simulink library "tqd"  (R2021b)
settings: Solver=VariableStepAuto  StartTime=0.0  StopTime=10.0  RelTol=1e-3
undefined symbols (not defined in the file): ATQD_AfterTqMinGain_X_Deg, ATQD_APSCreepBaseTqD_X_kph, ATQD_APSCreepBaseTqD_Y_Deg, ATQD_APSCreepBaseTqR_X_kph, ATQD_APSCreepBaseTqR_Y_Deg, ATQD_APSCreepIterm_X_kph, ATQD_APSCreepIterm_Y_kph, ATQD_APSCreepPterm_X_kph, ATQD_APSCreepPterm_Y_kph, ATQD_APSDecReq_X_kph, ATQD_APSDecReq_Y_mps2, ATQD_APSDecReqCMD_X_kph, ATQD_APSDecReqTs_X_pct, ATQD_APSDecTimeGain_X_Deg, ATQD_APSDecTimeGain_Y_s, ATQD_APSReqLowSpd_X_Deg, ATQD_AutoHoldReleaseBPS_X_Deg, ATQD_AWDLoadTrqnsGain_X_kg, ATQD_AWDLoadTrqnsGain_Y_pct, ATQD_BOSEnBPSPosn_X_kph, ATQD_BOSMap_X_rpm, ATQD_BOSMap_Y_pct, ATQD_CreepBaseTqD_X_kph, ATQD_CreepBaseTqD_Y_Deg, ATQD_CreepBaseTqR_X_kph, ATQD_CreepBaseTqR_Y_Deg, ATQD_CreepBPSDisPosn_X_Deg, ATQD_CreepBPSDisPosnR_X_Deg, ATQD_CreepBPSEnPosn_X_Deg, ATQD_CreepBPSEnPosnR_X_Deg, ATQD_CreepDeltaTq_X_kph, ATQD_CreepIterm_X_kph, ATQD_CreepIterm_Y_kph, ATQD_CreepItermMaxLimit_X_pct, ATQD_CreepPreloadTime_X_kph, ATQD_CreepPreloadTq_X_kph, ATQD_CreepPreloadTq_Y_s, ATQD_CreepProtTq_X_Deg, ATQD_CreepPterm_X_kph, ATQD_CreepPterm_Y_kph, ATQD_CreepRrTqSpRat_X_rpm, ATQD_CreepRrTqSpRat_Y_Nm, ATQD_CreepTargetSpdD_X_pct, ATQD_CreepTargetSpdR_X_pct, ATQD_ECOTqMapD_X_rpm, ATQD_ECOTqMapD_Y_pct, ATQD_EMTqMapD_X_rpm, ATQD_EMTqMapD_Y_pct, ATQD_EOPDTqMapDCon_X_rpm, ATQD_EOPDTqMapDCon_Y_Deg, ATQD_EscapeModePedTq_X_pct, ATQD_EscapeModePedTq_Y_rpm, ATQD_EscapeModePedTqFr_X_pct, ATQD_EscapeModePedTqFr_Y_rpm, ATQD_EstInitVehWeight_X_c, ATQD_FAfterTqCMDGain_X_rpm, ATQD_FAfterTqCMDGain_Y_pct, ATQD_FrLossMAPLowV_X_rpm, ATQD_FrLossMAPLowV_Y_Nm, ATQD_FrMotActReduce_X_rpm ... (+772)
libraries: simulink x211, hcu_lib x179, tqr x3
(part 24 of 28)

== system tqd/TQD/TorqueDemand/TorqueModule/DriverWhlTqDem/PedalMapWhlTq/NoLHM/ShiftD/LUT_D_ECO ==
  VTQD_TqTargetShaftSpd_rpm : Inport
  VTQD_ActAPSPosn_pct : Inport  Port=2
  VTQD_RegenMode_enum : Inport  Port=3
  VTQD_RollRegenEnable_flg : Inport  Port=4
  VTQD_RollingShaftSpd_rpm : Inport  Port=5
  VVMC_EstSlope_Deg : Inport  Port=6
  VTQD_APSReqTimer_s : Inport  Port=7
  VTQD_LowIdleAccPedal_flg : Inport  Port=8
  VTQD_OPDHoldEnRel_flg : Inport  Port=9
  VTQD_OPDHoldActRelTq_Nm : Inport  Port=10
  VTQD_VehActSpd_kph : Inport  Port=11
  VTQD_SlopeUp_flg : Inport  Port=12
  RegenTqMapDComp_bus : Inport  Port=13
  Action Port : ActionPort
  Bus Selector : BusSelector  OutputSignals=VTQD_RL1TqMapDComp_Nm,VTQD_RL2TqMapDComp_Nm,VTQD_RL3TqMapDComp_Nm,VTQD_RL4TqMapDComp_Nm,VTQD_RL5TqMapDComp_Nm
  Constant : Constant  Value=ENUM_REGENLEVEL_LV1
  Constant1 : Constant  Value=ENUM_REGENLEVEL_LV2
  Constant2 : Constant  Value=ENUM_REGENLEVEL_LV3
  Constant3 : Constant  Value=ENUM_REGENLEVEL_LV4
  Constant4 : Constant  Value=ENUM_REGENLEVEL_LV5
  Constant5 : Constant  Value=ENUM_REGENLEVEL_OPD
  ECO_Invalid_TqMap1 : Subsystem  TreatAsAtomicUnit=on
  ECO_Lv1_TqMap : Subsystem  TreatAsAtomicUnit=on
  ECO_Lv2_TqMap : Subsystem  TreatAsAtomicUnit=on
  ECO_Lv3_TqMap : Subsystem  TreatAsAtomicUnit=on
  ECO_Lv4_TqMap : Subsystem  TreatAsAtomicUnit=on
  ECO_Lv5_TqMap : Subsystem  TreatAsAtomicUnit=on
  ECO_OnePedal_TqMap : Subsystem  TreatAsAtomicUnit=on
  Equal{1..6} (6 alike) : RelationalOperator  Operator===  OutDataTypeStr=boolean  RndMeth=Simplest
  If : If  NumInputs=6  IfExpression=u1 ~= 0  ElseIfExpressions=u2 ~= 0, u3 ~= 0, u4 ~= 0, u5 ~= 0, u6 ~= 0
  MTQD_ECOTqMapD_Z_Nm : Lookup_n-D  BreakpointsForDimension1=ATQD_ECOTqMapD_Y_pct  BreakpointsForDimension2=ATQD_ECOTqMapD_X_rpm  Table=MTQD_ECOTqMapD_Z_Nm  ExtrapMethod=Clip  InternalRulePriority=Speed  RndMeth=Simplest  InputSameDT=on
      settings: InputPortMap=u0,u1
  MTQD_EL2TqMapD_Z_Nm : Lookup_n-D  BreakpointsForDimension1=ATQD_ECOTqMapD_Y_pct  BreakpointsForDimension2=ATQD_ECOTqMapD_X_rpm  Table=MTQD_EL2TqMapD_Z_Nm  ExtrapMethod=Clip  InternalRulePriority=Speed  RndMeth=Simplest  InputSameDT=on
      settings: InputPortMap=u0,u1
  MTQD_EL3TqMapD_Z_Nm : Lookup_n-D  BreakpointsForDimension1=ATQD_ECOTqMapD_Y_pct  BreakpointsForDimension2=ATQD_ECOTqMapD_X_rpm  Table=MTQD_EL3TqMapD_Z_Nm  ExtrapMethod=Clip  InternalRulePriority=Speed  RndMeth=Simplest  InputSameDT=on
      settings: InputPortMap=u0,u1
  MTQD_EL4TqMapD_Z_Nm : Lookup_n-D  BreakpointsForDimension1=ATQD_ECOTqMapD_Y_pct  BreakpointsForDimension2=ATQD_ECOTqMapD_X_rpm  Table=MTQD_EL4TqMapD_Z_Nm  ExtrapMethod=Clip  InternalRulePriority=Speed  RndMeth=Simplest  InputSameDT=on
      settings: InputPortMap=u0,u1
  MTQD_EL5TqMapD_Z_Nm : Lookup_n-D  BreakpointsForDimension1=ATQD_ECOTqMapD_Y_pct  BreakpointsForDimension2=ATQD_ECOTqMapD_X_rpm  Table=MTQD_EL5TqMapD_Z_Nm  ExtrapMethod=Clip  InternalRulePriority=Speed  RndMeth=Simplest  InputSameDT=on
      settings: InputPortMap=u0,u1
  MTQD_EOPDTqMapDCon_Z_Nm : Lookup_n-D  BreakpointsForDimension1=ATQD_EOPDTqMapDCon_Y_Deg  BreakpointsForDimension2=ATQD_EOPDTqMapDCon_X_rpm  Table=MTQD_EOPDTqMapDCon_Z_Nm  ExtrapMethod=Clip  InternalRulePriority=Speed  RndMeth=Simplest  InputSameDT=on
      settings: InputPortMap=u0,u1
  MTQD_EOPDTqMapD_Z_Nm : Lookup_n-D  BreakpointsForDimension1=ATQD_ECOTqMapD_Y_pct  BreakpointsForDimension2=ATQD_ECOTqMapD_X_rpm  Table=MTQD_EOPDTqMapD_Z_Nm  ExtrapMethod=Clip  InternalRulePriority=Speed  RndMeth=Simplest  InputSameDT=on
      settings: InputPortMap=u0,u1
  MTQD_RollGenMapEL1_Z_Nm : Lookup_n-D  BreakpointsForDimension1=ATQD_RollGenMapEL1_Y_rpm  BreakpointsForDimension2=ATQD_RollGenMapEL1_X_rpm  Table=MTQD_RollGenMapEL1_Z_Nm  ExtrapMethod=Clip  InternalRulePriority=Speed  RndMeth=Simplest  InputSameDT=on
      settings: InputPortMap=u0,u1
  Merge : Merge  Inputs=7
  VTQD_WhlTqECOD_Nm : Outport
  wires:
  [VTQD_ECOTqMapD_Nm] -> ECO_Lv1_TqMap/3(MTQD_ECOTqMapD_Z_Nm)
  [VTQD_RollGenMapEL1_Nm] -> ECO_Lv1_TqMap/2(MTQD_RollGenMapEL1_Z_Nm)
  [VTQD_RollRegenEnable_flg] -> ECO_Lv1_TqMap/1(VTQD_RollRegenEnable_flg)
  [VTQD_TqTargetShaftSpd_rpm] -> MTQD_RollGenMapEL1_Z_Nm/2
  [VTQD_RollingShaftSpd_rpm] -> MTQD_RollGenMapEL1_Z_Nm/1
  MTQD_RollGenMapEL1_Z_Nm/1 -> [VTQD_RollGenMapEL1_Nm]
  VTQD_RollingShaftSpd_rpm/1 -> [VTQD_RollingShaftSpd_rpm]
  VTQD_RollRegenEnable_flg/1 -> [VTQD_RollRegenEnable_flg]
  Equal6/1 -> If/6
  [VTQD_RegenMode_enum] -> Equal6/1
  Constant5/1 -> Equal6/2
  Equal5/1 -> If/5
  [VTQD_RegenMode_enum] -> Equal5/1
  Constant4/1 -> Equal5/2
  Equal4/1 -> If/4
  [VTQD_RegenMode_enum] -> Equal4/1
  Constant3/1 -> Equal4/2
  [VTQD_RegenMode_enum] -> Equal3/1
  Constant2/1 -> Equal3/2
  [VTQD_RegenMode_enum] -> Equal2/1
  Constant1/1 -> Equal2/2
  Constant/1 -> Equal1/2
  [VTQD_RegenMode_enum] -> Equal1/1
  [VTQD_EOPDTqMapD_Nm] -> ECO_OnePedal_TqMap/1(VTQD_EOPDTqMapDIn_Nm)
  If/6 -> ECO_OnePedal_TqMap/Action
  ECO_OnePedal_TqMap/1(VTQD_EOPDTqMapDOut_Nm) -> Merge/6
  [VTQD_EL5TqMapD_Nm] -> ECO_Lv5_TqMap/1(VTQD_EL5TqMapDIn_Nm)
  If/5 -> ECO_Lv5_TqMap/Action
  ECO_Lv5_TqMap/1(VTQD_EL5TqMapDOut_Nm) -> Merge/5
  ECO_Lv4_TqMap/1(VTQD_EL4TqMapDOut_Nm) -> Merge/4
  If/4 -> ECO_Lv4_TqMap/Action
  [VTQD_EL4TqMapD_Nm] -> ECO_Lv4_TqMap/1(VTQD_EL4TqMapDIn_Nm)
  [VTQD_EL3TqMapD_Nm] -> ECO_Lv3_TqMap/1(VTQD_EL3TqMapDIn_Nm)
  If/3 -> ECO_Lv3_TqMap/Action
  ECO_Lv3_TqMap/1(VTQD_EL3TqMapDOut_Nm) -> Merge/3
  [VTQD_EL2TqMapD_Nm] -> ECO_Lv2_TqMap/1(VTQD_EL2TqMapDIn_Nm)
  ECO_Lv2_TqMap/1(VTQD_EL2TqMapDOut_Nm) -> Merge/2
  If/2 -> ECO_Lv2_TqMap/Action
  ECO_Lv1_TqMap/1(VTQD_EL1TqMapDOut_Nm) -> Merge/1
  Equal1/1 -> If/1
  Equal2/1 -> If/2
  If/1 -> ECO_Lv1_TqMap/Action
  Merge/1 -> VTQD_WhlTqECOD_Nm/1
  Equal3/1 -> If/3
  [VTQD_TqTargetShaftSpd_rpm] -> MTQD_EOPDTqMapD_Z_Nm/2
  [VTQD_ActAPSPosn_pct] -> MTQD_EOPDTqMapD_Z_Nm/1
  [VTQD_TqTargetShaftSpd_rpm] -> MTQD_EL5TqMapD_Z_Nm/2
  [VTQD_ActAPSPosn_pct] -> MTQD_EL5TqMapD_Z_Nm/1
  [VTQD_TqTargetShaftSpd_rpm] -> MTQD_EL3TqMapD_Z_Nm/2
  [VTQD_ActAPSPosn_pct] -> MTQD_EL3TqMapD_Z_Nm/1
  [VTQD_TqTargetShaftSpd_rpm] -> MTQD_EL2TqMapD_Z_Nm/2
  [VTQD_ActAPSPosn_pct] -> MTQD_EL2TqMapD_Z_Nm/1
  MTQD_EL5TqMapD_Z_Nm/1 -> [VTQD_EL5TqMapD_Nm]
  MTQD_EL4TqMapD_Z_Nm/1 -> [VTQD_EL4TqMapD_Nm]
  [VTQD_TqTargetShaftSpd_rpm] -> MTQD_EL4TqMapD_Z_Nm/2
  [VTQD_ActAPSPosn_pct] -> MTQD_EL4TqMapD_Z_Nm/1
  MTQD_EOPDTqMapD_Z_Nm/1 -> [VTQD_EOPDTqMapD_Nm]
  MTQD_EL3TqMapD_Z_Nm/1 -> [VTQD_EL3TqMapD_Nm]
  MTQD_EL2TqMapD_Z_Nm/1 -> [VTQD_EL2TqMapD_Nm]
  [VTQD_ActAPSPosn_pct] -> MTQD_ECOTqMapD_Z_Nm/1
  [VTQD_TqTargetShaftSpd_rpm] -> MTQD_ECOTqMapD_Z_Nm/2
  VTQD_RegenMode_enum/1 -> [VTQD_RegenMode_enum]
  VTQD_ActAPSPosn_pct/1 -> [VTQD_ActAPSPosn_pct]
  VTQD_TqTargetShaftSpd_rpm/1 -> [VTQD_TqTargetShaftSpd_rpm]
  MTQD_ECOTqMapD_Z_Nm/1 -> [VTQD_ECOTqMapD_Nm]
  ECO_Invalid_TqMap1/1(VTQD_EL1TqMapDOut_Nm) -> Merge/7
  [VTQD_RollRegenEnable_flg] -> ECO_Invalid_TqMap1/1(VTQD_RollRegenEnable_flg)
  [VTQD_RollGenMapEL1_Nm] -> ECO_Invalid_TqMap1/2(MTQD_RollGenMapEL1_Z_Nm)
  [VTQD_ECOTqMapD_Nm] -> ECO_Invalid_TqMap1/3(MTQD_ECOTqMapD_Z_Nm)
  If/7 -> ECO_Invalid_TqMap1/Action
  [VTQD_TqTargetShaftSpd_rpm] -> MTQD_EOPDTqMapDCon_Z_Nm/2
  [VVMC_EstSlope_Deg] -> MTQD_EOPDTqMapDCon_Z_Nm/1
  MTQD_EOPDTqMapDCon_Z_Nm/1 -> [VTQD_EOPDTqMapDCon_Nm]
  VVMC_EstSlope_Deg/1 -> [VVMC_EstSlope_Deg]
  VTQD_APSReqTimer_s/1 -> [VTQD_APSReqTimer_s]
  [VTQD_EOPDTqMapDCon_Nm] -> ECO_OnePedal_TqMap/2(VTQD_EOPDTqMapDCon_Nm)
  [VTQD_APSReqTimer_s] -> ECO_OnePedal_TqMap/3(VTQD_APSReqTimer_s)
  [VTQD_LowIdleAccPedal_flg] -> ECO_OnePedal_TqMap/4(VTQD_LowIdleAccPedal_flg)
  VTQD_LowIdleAccPedal_flg/1 -> [VTQD_LowIdleAccPedal_flg]
  VTQD_OPDHoldActRelTq_Nm/1 -> [VTQD_OPDHoldActRelTq_Nm]
  VTQD_OPDHoldEnRel_flg/1 -> [VTQD_OPDHoldEnRel_flg]
  VTQD_VehActSpd_kph/1 -> [VTQD_VehActSpd_kph]
  [VTQD_VehActSpd_kph] -> ECO_OnePedal_TqMap/7(VTQD_VehActSpd_kph)
  [VTQD_OPDHoldActRelTq_Nm] -> ECO_OnePedal_TqMap/6(VTQD_OPDHoldActRelTq_Nm)
  [VTQD_OPDHoldEnRel_flg] -> ECO_OnePedal_TqMap/5(VTQD_OPDHoldEnRel_flg)
  VTQD_SlopeUp_flg/1 -> [VTQD_SlopeUp_flg]
  [VTQD_SlopeUp_flg] -> ECO_OnePedal_TqMap/8(VTQD_SlopeUp_flg)
  [VTQD_ActAPSPosn_pct] -> ECO_OnePedal_TqMap/9(VTQD_ActAPSPosn_pct)
  RegenTqMapDComp_bus/1 -> [RegenTqMapDComp_bus]
  [RegenTqMapDComp_bus] -> Bus Selector/1
  Bus Selector/4 -> [VTQD_RL4TqMapDComp_Nm]  "<VTQD_RL4TqMapDComp_Nm>"
  Bus Selector/1 -> [VTQD_RL1TqMapDComp_Nm]  "<VTQD_RL1TqMapDComp_Nm>"
  Bus Selector/2 -> [VTQD_RL2TqMapDComp_Nm]  "<VTQD_RL2TqMapDComp_Nm>"
  Bus Selector/3 -> [VTQD_RL3TqMapDComp_Nm]  "<VTQD_RL3TqMapDComp_Nm>"
  Bus Selector/5 -> [VTQD_RL5TqMapDComp_Nm]  "<VTQD_RL5TqMapDComp_Nm>"
  [VTQD_RL1TqMapDComp_Nm] -> ECO_Lv1_TqMap/4(VTQD_RL1TqMapDComp_Nm)
  [VTQD_RL2TqMapDComp_Nm] -> ECO_Lv2_TqMap/2(VTQD_RL2TqMapDComp_Nm)
  [VTQD_RL3TqMapDComp_Nm] -> ECO_Lv3_TqMap/2(VTQD_RL3TqMapDComp_Nm)
  [VTQD_RL4TqMapDComp_Nm] -> ECO_Lv4_TqMap/2(VTQD_RL4TqMapDComp_Nm)
  [VTQD_RL5TqMapDComp_Nm] -> ECO_Lv5_TqMap/2(VTQD_RL5TqMapDComp_Nm)

== system tqd/TQD/TorqueDemand/TorqueModule/DriverWhlTqDem/PedalMapWhlTq/NoLHM/ShiftD/LUT_D_EscapeMode ==
  VTQD_TqTargetShaftSpd_rpm : Inport
  VTQD_ActAPSPosn_pct : Inport  Port=2
  Action Port : ActionPort
  MTQD_EMTqMapD_Z_Nm : Lookup_n-D  BreakpointsForDimension1=ATQD_EMTqMapD_Y_pct  BreakpointsForDimension2=ATQD_EMTqMapD_X_rpm  Table=MTQD_EMTqMapD_Z_Nm  ExtrapMethod=Clip  InternalRulePriority=Speed  RndMeth=Simplest  InputSameDT=on
      settings: InputPortMap=u0,u1
  VTQD_WhlTqEscapeMode_Nm : Outport
  wires:
  [VTQD_ActAPSPosn_pct] -> MTQD_EMTqMapD_Z_Nm/1
  [VTQD_TqTargetShaftSpd_rpm] -> MTQD_EMTqMapD_Z_Nm/2
  VTQD_ActAPSPosn_pct/1 -> [VTQD_ActAPSPosn_pct]
  VTQD_TqTargetShaftSpd_rpm/1 -> [VTQD_TqTargetShaftSpd_rpm]
  MTQD_EMTqMapD_Z_Nm/1 -> VTQD_WhlTqEscapeMode_Nm/1

== system tqd/TQD/TorqueDemand/TorqueModule/DriverWhlTqDem/PedalMapWhlTq/NoLHM/ShiftD/LUT_D_Normal ==
  VTQD_TqTargetShaftSpd_rpm : Inport
  VTQD_ActAPSPosn_pct : Inport  Port=2
  VTQD_RegenMode_enum : Inport  Port=3
  VVMC_EstSlope_Deg : Inport  Port=4
  VTQD_APSReqTimer_s : Inport  Port=5
  VTQD_LowIdleAccPedal_flg : Inport  Port=6
  VTQD_OPDHoldEnRel_flg : Inport  Port=7
  VTQD_OPDHoldActRelTq_Nm : Inport  Port=8
  VTQD_VehActSpd_kph : Inport  Port=9
  VTQD_SlopeUp_flg : Inport  Port=10
  RegenTqMapDComp_bus : Inport  Port=11
  Action Port : ActionPort
  Bus Selector : BusSelector  OutputSignals=VTQD_RL1TqMapDComp_Nm,VTQD_RL2TqMapDComp_Nm,VTQD_RL3TqMapDComp_Nm,VTQD_RL4TqMapDComp_Nm,VTQD_RL5TqMapDComp_Nm
  Constant : Constant  Value=ENUM_REGENLEVEL_LV1
  Constant1 : Constant  Value=ENUM_REGENLEVEL_LV2
  Constant2 : Constant  Value=ENUM_REGENLEVEL_LV3
  Constant3 : Constant  Value=ENUM_REGENLEVEL_LV4
  Constant4 : Constant  Value=ENUM_REGENLEVEL_LV5
  Constant5 : Constant  Value=ENUM_REGENLEVEL_OPD
  Equal{1..6} (6 alike) : RelationalOperator  Operator===  OutDataTypeStr=boolean  RndMeth=Simplest
  If : If  NumInputs=6  IfExpression=u1 ~= 0  ElseIfExpressions=u2 ~= 0, u3 ~= 0, u4 ~= 0, u5 ~= 0, u6~=0
  MTQD_NL1TqMapD_Z_Nm : Lookup_n-D  BreakpointsForDimension1=ATQD_NL1TqMapD_Y_pct  BreakpointsForDimension2=ATQD_NL1TqMapD_X_rpm  Table=MTQD_NL1TqMapD_Z_Nm  ExtrapMethod=Clip  InternalRulePriority=Speed  RndMeth=Simplest  InputSameDT=on
      settings: InputPortMap=u0,u1
  MTQD_NL2TqMapD_Z_Nm : Lookup_n-D  BreakpointsForDimension1=ATQD_NL1TqMapD_Y_pct  BreakpointsForDimension2=ATQD_NL1TqMapD_X_rpm  Table=MTQD_NL2TqMapD_Z_Nm  ExtrapMethod=Clip  InternalRulePriority=Speed  RndMeth=Simplest  InputSameDT=on
      settings: InputPortMap=u0,u1
  MTQD_NL3TqMapD_Z_Nm : Lookup_n-D  BreakpointsForDimension1=ATQD_NL1TqMapD_Y_pct  BreakpointsForDimension2=ATQD_NL1TqMapD_X_rpm  Table=MTQD_NL3TqMapD_Z_Nm  ExtrapMethod=Clip  InternalRulePriority=Speed  RndMeth=Simplest  InputSameDT=on
      settings: InputPortMap=u0,u1
  MTQD_NL4TqMapD_Z_Nm1 : Lookup_n-D  BreakpointsForDimension1=ATQD_NL1TqMapD_Y_pct  BreakpointsForDimension2=ATQD_NL1TqMapD_X_rpm  Table=MTQD_NL4TqMapD_Z_Nm  ExtrapMethod=Clip  InternalRulePriority=Speed  RndMeth=Simplest  InputSameDT=on
      settings: InputPortMap=u0,u1
  MTQD_NL5TqMapD_Z_Nm1 : Lookup_n-D  BreakpointsForDimension1=ATQD_NL1TqMapD_Y_pct  BreakpointsForDimension2=ATQD_NL1TqMapD_X_rpm  Table=MTQD_NL5TqMapD_Z_Nm  ExtrapMethod=Clip  InternalRulePriority=Speed  RndMeth=Simplest  InputSameDT=on
      settings: InputPortMap=u0,u1
  MTQD_NOPDTqMapDCon_Z_Nm : Lookup_n-D  BreakpointsForDimension1=ATQD_NOPDTqMapDCon_Y_Deg  BreakpointsForDimension2=ATQD_NOPDTqMapDCon_X_rpm  Table=MTQD_NOPDTqMapDCon_Z_Nm  ExtrapMethod=Clip  InternalRulePriority=Speed  RndMeth=Simplest  InputSameDT=on
      settings: InputPortMap=u0,u1
  MTQD_NOPDTqMapD_Z_Nm1 : Lookup_n-D  BreakpointsForDimension1=ATQD_NL1TqMapD_Y_pct  BreakpointsForDimension2=ATQD_NL1TqMapD_X_rpm  Table=MTQD_NOPDTqMapD_Z_Nm  ExtrapMethod=Clip  InternalRulePriority=Speed  RndMeth=Simplest  InputSameDT=on
      settings: InputPortMap=u0,u1
  Merge : Merge  Inputs=7
  NRM_Invalid_TqMap1 : Subsystem  TreatAsAtomicUnit=on
  NRM_Lv1_TqMap : Subsystem  TreatAsAtomicUnit=on
  NRM_Lv2_TqMap : Subsystem  TreatAsAtomicUnit=on
  NRM_Lv3_TqMap : Subsystem  TreatAsAtomicUnit=on
  NRM_Lv4_TqMap : Subsystem  TreatAsAtomicUnit=on
  NRM_Lv5_TqMap : Subsystem  TreatAsAtomicUnit=on
  NRM_OnePedal_TqMap : Subsystem  TreatAsAtomicUnit=on
  VTQD_WhlTqNRMD_Nm : Outport
  wires:
  Equal6/1 -> If/6
  [VTQD_RegenMode_enum] -> Equal6/1
  Constant5/1 -> Equal6/2
  Equal5/1 -> If/5
  [VTQD_RegenMode_enum] -> Equal5/1
  Constant4/1 -> Equal5/2
  Equal4/1 -> If/4
  [VTQD_RegenMode_enum] -> Equal4/1
  Constant3/1 -> Equal4/2
  [VTQD_RegenMode_enum] -> Equal3/1
  Constant2/1 -> Equal3/2
  [VTQD_RegenMode_enum] -> Equal2/1
  Constant1/1 -> Equal2/2
  Constant/1 -> Equal1/2
  [VTQD_RegenMode_enum] -> Equal1/1
  If/6 -> NRM_OnePedal_TqMap/Action
  NRM_OnePedal_TqMap/1(VTQD_NOPDTqMapDOut_Nm) -> Merge/6
  [VTQD_NL5TqMapD_Nm] -> NRM_Lv5_TqMap/1(VTQD_NL5TqMapDIn_Nm)
  If/5 -> NRM_Lv5_TqMap/Action
  NRM_Lv5_TqMap/1(VTQD_NL5TqMapDOut_Nm) -> Merge/5
  NRM_Lv4_TqMap/1(VTQD_NL4TqMapDOut_Nm) -> Merge/4
  If/4 -> NRM_Lv4_TqMap/Action
  [VTQD_NL4TqMapD_Nm] -> NRM_Lv4_TqMap/1(VTQD_NL4TqMapDIn_Nm)
  [VTQD_NL3TqMapD_Nm] -> NRM_Lv3_TqMap/1(VTQD_NL3TqMapDIn_Nm)
  If/3 -> NRM_Lv3_TqMap/Action
  NRM_Lv3_TqMap/1(VTQD_NL3TqMapDOut_Nm) -> Merge/3
  [VTQD_NL2TqMapD_Nm] -> NRM_Lv2_TqMap/1(VTQD_NL2TqMapDIn_Nm)
  NRM_Lv2_TqMap/1(VTQD_NL2TqMapDOut_Nm) -> Merge/2
  If/2 -> NRM_Lv2_TqMap/Action
  NRM_Lv1_TqMap/1(VTQD_NL1TqMapDOut_Nm) -> Merge/1
  [VTQD_NL1TqMapD_Nm] -> NRM_Lv1_TqMap/1(VTQD_NL1TqMapDIn_Nm)
  Equal1/1 -> If/1
  Equal2/1 -> If/2
  If/1 -> NRM_Lv1_TqMap/Action
  Merge/1 -> VTQD_WhlTqNRMD_Nm/1
  Equal3/1 -> If/3
  [VTQD_TqTargetShaftSpd_rpm] -> MTQD_NOPDTqMapD_Z_Nm1/2
  [VTQD_ActAPSPosn_pct] -> MTQD_NOPDTqMapD_Z_Nm1/1
  [VTQD_TqTargetShaftSpd_rpm] -> MTQD_NL5TqMapD_Z_Nm1/2
  [VTQD_ActAPSPosn_pct] -> MTQD_NL5TqMapD_Z_Nm1/1
  [VTQD_TqTargetShaftSpd_rpm] -> MTQD_NL3TqMapD_Z_Nm/2
  [VTQD_ActAPSPosn_pct] -> MTQD_NL3TqMapD_Z_Nm/1
  [VTQD_TqTargetShaftSpd_rpm] -> MTQD_NL2TqMapD_Z_Nm/2
  [VTQD_ActAPSPosn_pct] -> MTQD_NL2TqMapD_Z_Nm/1
  MTQD_NL5TqMapD_Z_Nm1/1 -> [VTQD_NL5TqMapD_Nm]
  MTQD_NL4TqMapD_Z_Nm1/1 -> [VTQD_NL4TqMapD_Nm]
  [VTQD_TqTargetShaftSpd_rpm] -> MTQD_NL4TqMapD_Z_Nm1/2
  [VTQD_ActAPSPosn_pct] -> MTQD_NL4TqMapD_Z_Nm1/1
  MTQD_NOPDTqMapD_Z_Nm1/1 -> [VTQD_NOPDTqMapD_Nm]
  MTQD_NL3TqMapD_Z_Nm/1 -> [VTQD_NL3TqMapD_Nm]
  MTQD_NL2TqMapD_Z_Nm/1 -> [VTQD_NL2TqMapD_Nm]
  [VTQD_ActAPSPosn_pct] -> MTQD_NL1TqMapD_Z_Nm/1
  [VTQD_TqTargetShaftSpd_rpm] -> MTQD_NL1TqMapD_Z_Nm/2
  VTQD_RegenMode_enum/1 -> [VTQD_RegenMode_enum]
  VTQD_ActAPSPosn_pct/1 -> [VTQD_ActAPSPosn_pct]
  VTQD_TqTargetShaftSpd_rpm/1 -> [VTQD_TqTargetShaftSpd_rpm]
  MTQD_NL1TqMapD_Z_Nm/1 -> [VTQD_NL1TqMapD_Nm]
  [VTQD_NL1TqMapD_Nm] -> NRM_Invalid_TqMap1/1(VTQD_NL1TqMapDIn_Nm)
  If/7 -> NRM_Invalid_TqMap1/Action
  NRM_Invalid_TqMap1/1(VTQD_NL1TqMapDOut_Nm) -> Merge/7
  [VTQD_TqTargetShaftSpd_rpm] -> MTQD_NOPDTqMapDCon_Z_Nm/2
  [VVMC_EstSlope_Deg] -> MTQD_NOPDTqMapDCon_Z_Nm/1
  MTQD_NOPDTqMapDCon_Z_Nm/1 -> [VTQD_NOPDTqMapDCon_Nm]
  VVMC_EstSlope_Deg/1 -> [VVMC_EstSlope_Deg]
  [VTQD_APSReqTimer_s] -> NRM_OnePedal_TqMap/3(VTQD_APSReqTimer_s)
  VTQD_APSReqTimer_s/1 -> [VTQD_APSReqTimer_s]
  [VTQD_LowIdleAccPedal_flg] -> NRM_OnePedal_TqMap/4(VTQD_LowIdleAccPedal_flg)
  VTQD_LowIdleAccPedal_flg/1 -> [VTQD_LowIdleAccPedal_flg]
  VTQD_OPDHoldEnRel_flg/1 -> [VTQD_OPDHoldEnRel_flg]
  VTQD_OPDHoldActRelTq_Nm/1 -> [VTQD_OPDHoldActRelTq_Nm]
  VTQD_VehActSpd_kph/1 -> [VTQD_VehActSpd_kph]
  [VTQD_OPDHoldEnRel_flg] -> NRM_OnePedal_TqMap/5(VTQD_OPDHoldEnRel_flg)
  [VTQD_OPDHoldActRelTq_Nm] -> NRM_OnePedal_TqMap/6(VTQD_OPDHoldActRelTq_Nm)
  [VTQD_VehActSpd_kph] -> NRM_OnePedal_TqMap/7(VTQD_VehActSpd_kph)
  VTQD_SlopeUp_flg/1 -> [VTQD_SlopeUp_flg]
  [VTQD_SlopeUp_flg] -> NRM_OnePedal_TqMap/8(VTQD_SlopeUp_flg)
  [VTQD_NOPDTqMapD_Nm] -> NRM_OnePedal_TqMap/1(VTQD_NOPDTqMapDIn_Nm)
  [VTQD_NOPDTqMapDCon_Nm] -> NRM_OnePedal_TqMap/2(VTQD_NOPDTqMapDCon_Nm)
  [VTQD_ActAPSPosn_pct] -> NRM_OnePedal_TqMap/9(VTQD_ActAPSPosn_pct)
  RegenTqMapDComp_bus/1 -> [RegenTqMapDComp_bus]
  [RegenTqMapDComp_bus] -> Bus Selector/1
  Bus Selector/1 -> [VTQD_RL1TqMapDComp_Nm]  "<VTQD_RL1TqMapDComp_Nm>"
  Bus Selector/2 -> [VTQD_RL2TqMapDComp_Nm]  "<VTQD_RL2TqMapDComp_Nm>"
  Bus Selector/3 -> [VTQD_RL3TqMapDComp_Nm]  "<VTQD_RL3TqMapDComp_Nm>"
  Bus Selector/4 -> [VTQD_RL4TqMapDComp_Nm]  "<VTQD_RL4TqMapDComp_Nm>"
  Bus Selector/5 -> [VTQD_RL5TqMapDComp_Nm]  "<VTQD_RL5TqMapDComp_Nm>"
  [VTQD_RL1TqMapDComp_Nm] -> NRM_Lv1_TqMap/2(VTQD_RL1TqMapDComp_Nm)
  [VTQD_RL2TqMapDComp_Nm] -> NRM_Lv2_TqMap/2(VTQD_RL2TqMapDComp_Nm)
  [VTQD_RL3TqMapDComp_Nm] -> NRM_Lv3_TqMap/2(VTQD_RL3TqMapDComp_Nm)
  [VTQD_RL4TqMapDComp_Nm] -> NRM_Lv4_TqMap/2(VTQD_RL4TqMapDComp_Nm)
  [VTQD_RL5TqMapDComp_Nm] -> NRM_Lv5_TqMap/2(VTQD_RL5TqMapDComp_Nm)

== system tqd/TQD/TorqueDemand/TorqueModule/DriverWhlTqDem/PedalMapWhlTq/NoLHM/ShiftD/LUT_D_SnowMode ==
  VTQD_TqTargetShaftSpd_rpm : Inport
  VTQD_ActAPSPosn_pct : Inport  Port=2
  VTQD_RegenMode_enum : Inport  Port=3
  VTQD_PreDecTqLowLim_Nm : Inport  Port=4
  Action Port : ActionPort
  Constant1 : Constant  Value=ZERO_FLOAT
  Constant2 : Constant  Value=ENUM_REGENLEVEL_LV1
  Constant3 : Constant  Value=KTQD_PedalMapRDCUpLim_Nm
  Equal : RelationalOperator  Operator===  OutDataTypeStr=boolean  RndMeth=Simplest
  MTQD_SN1TqMapD_Z_Nm : Lookup_n-D  BreakpointsForDimension1=ATQD_SNTqMapD_Y_pct  BreakpointsForDimension2=ATQD_SNTqMapD_X_rpm  Table=MTQD_SNTqMapD_Z_Nm  ExtrapMethod=Clip  InternalRulePriority=Speed  RndMeth=Simplest  InputSameDT=on
      settings: InputPortMap=u0,u1
  Saturation Dynamic : simulink/Discontinuities/Saturation Dynamic  OutMin=[]  OutMax=[]  OutDataTypeStr=Inherit: Same as second input  OutDataType=fixdt(1, 16)  OutScaling=2^-10  DoSatur=off
  Switch : Switch  Criteria=u2 > Threshold
  VTQD_WhlTqSnowMode_Nm : Outport
  wires:
  VTQD_TqTargetShaftSpd_rpm/1 -> [VTQD_TqTargetShaftSpd_rpm]
  VTQD_ActAPSPosn_pct/1 -> [VTQD_ActAPSPosn_pct]
  VTQD_RegenMode_enum/1 -> [VTQD_RegenMode_enum]
  MTQD_SN1TqMapD_Z_Nm/1 -> [VTQD_SNTqMapD_Nm]  "VTQD_SNTqMapD_Nm"
  [VTQD_RegenMode_enum] -> Equal/1
  Equal/1 -> Switch/2
  Constant2/1 -> Equal/2
  [VTQD_ActAPSPosn_pct] -> MTQD_SN1TqMapD_Z_Nm/1
  [VTQD_TqTargetShaftSpd_rpm] -> MTQD_SN1TqMapD_Z_Nm/2
  Constant1/1 -> Switch/1
  Constant3/1 -> Saturation Dynamic/1
  VTQD_PreDecTqLowLim_Nm/1 -> [VTQD_PreDecTqLowLim_Nm]
  [VTQD_SNTqMapD_Nm] -> Saturation Dynamic/2
  [VTQD_PreDecTqLowLim_Nm] -> Switch/3
  Switch/1 -> Saturation Dynamic/3
  Saturation Dynamic/1 -> VTQD_WhlTqSnowMode_Nm/1

== system tqd/TQD/TorqueDemand/TorqueModule/DriverWhlTqDem/PedalMapWhlTq/NoLHM/ShiftD/LUT_D_Sport ==
  VTQD_TqTargetShaftSpd_rpm : Inport
  VTQD_ActAPSPosn_pct : Inport  Port=2
  VTQD_RegenMode_enum : Inport  Port=3
  VVMC_EstSlope_Deg : Inport  Port=4
  VTQD_APSReqTimer_s : Inport  Port=5
  VTQD_LowIdleAccPedal_flg : Inport  Port=6
  VTQD_OPDHoldEnRel_flg : Inport  Port=7
  VTQD_OPDHoldActRelTq_Nm : Inport  Port=8
  VTQD_VehActSpd_kph : Inport  Port=9
  VTQD_SlopeUp_flg : Inport  Port=10
  RegenTqMapDComp_bus : Inport  Port=11
  Action Port : ActionPort
  Bus Selector : BusSelector  OutputSignals=VTQD_RL1TqMapDComp_Nm,VTQD_RL2TqMapDComp_Nm,VTQD_RL3TqMapDComp_Nm,VTQD_RL4TqMapDComp_Nm,VTQD_RL5TqMapDComp_Nm
  Constant : Constant  Value=ENUM_REGENLEVEL_LV1
  Constant1 : Constant  Value=ENUM_REGENLEVEL_LV2
  Constant2 : Constant  Value=ENUM_REGENLEVEL_LV3
  Constant3 : Constant  Value=ENUM_REGENLEVEL_LV4
  Constant4 : Constant  Value=ENUM_REGENLEVEL_LV5
  Constant5 : Constant  Value=ENUM_REGENLEVEL_OPD
  Equal{1..6} (6 alike) : RelationalOperator  Operator===  OutDataTypeStr=boolean  RndMeth=Simplest
  If : If  NumInputs=6  IfExpression=u1 ~= 0  ElseIfExpressions=u2 ~= 0, u3 ~= 0, u4 ~= 0, u5 ~= 0, u6 ~= 0
  MTQD_SL1TqMapD_Z_Nm : Lookup_n-D  BreakpointsForDimension1=ATQD_SL1TqMapD_Y_pct  BreakpointsForDimension2=ATQD_SL1TqMapD_X_rpm  Table=MTQD_SL1TqMapD_Z_Nm  ExtrapMethod=Clip  InternalRulePriority=Speed  RndMeth=Simplest  InputSameDT=on
      settings: InputPortMap=u0,u1
  MTQD_SL2TqMapD_Z_Nm : Lookup_n-D  BreakpointsForDimension1=ATQD_SL1TqMapD_Y_pct  BreakpointsForDimension2=ATQD_SL1TqMapD_X_rpm  Table=MTQD_SL2TqMapD_Z_Nm  ExtrapMethod=Clip  InternalRulePriority=Speed  RndMeth=Simplest  InputSameDT=on
      settings: InputPortMap=u0,u1
  MTQD_SL3TqMapD_Z_Nm : Lookup_n-D  BreakpointsForDimension1=ATQD_SL1TqMapD_Y_pct  BreakpointsForDimension2=ATQD_SL1TqMapD_X_rpm  Table=MTQD_SL3TqMapD_Z_Nm  ExtrapMethod=Clip  InternalRulePriority=Speed  RndMeth=Simplest  InputSameDT=on
      settings: InputPortMap=u0,u1
  MTQD_SL4TqMapD_Z_Nm : Lookup_n-D  BreakpointsForDimension1=ATQD_SL1TqMapD_Y_pct  BreakpointsForDimension2=ATQD_SL1TqMapD_X_rpm  Table=MTQD_SL4TqMapD_Z_Nm  ExtrapMethod=Clip  InternalRulePriority=Speed  RndMeth=Simplest  InputSameDT=on
      settings: InputPortMap=u0,u1
  MTQD_SL5TqMapD_Z_Nm : Lookup_n-D  BreakpointsForDimension1=ATQD_SL1TqMapD_Y_pct  BreakpointsForDimension2=ATQD_SL1TqMapD_X_rpm  Table=MTQD_SL5TqMapD_Z_Nm  ExtrapMethod=Clip  InternalRulePriority=Speed  RndMeth=Simplest  InputSameDT=on
      settings: InputPortMap=u0,u1
  MTQD_SOPDTqMapDCon_Z_Nm : Lookup_n-D  BreakpointsForDimension1=ATQD_SOPDTqMapDCon_Y_Deg  BreakpointsForDimension2=ATQD_SOPDTqMapDCon_X_rpm  Table=MTQD_SOPDTqMapDCon_Z_Nm  ExtrapMethod=Clip  InternalRulePriority=Speed  RndMeth=Simplest  InputSameDT=on
      settings: InputPortMap=u0,u1
  MTQD_SOPDTqMapD_Z_Nm : Lookup_n-D  BreakpointsForDimension1=ATQD_SL1TqMapD_Y_pct  BreakpointsForDimension2=ATQD_SL1TqMapD_X_rpm  Table=MTQD_SOPDTqMapD_Z_Nm  ExtrapMethod=Clip  InternalRulePriority=Speed  RndMeth=Simplest  InputSameDT=on
      settings: InputPortMap=u0,u1
  Merge : Merge  Inputs=7
  Sport_Invalid_TqMap1 : Subsystem  TreatAsAtomicUnit=on
  Sport_Lv1_TqMap : Subsystem  TreatAsAtomicUnit=on
  Sport_Lv2_TqMap : Subsystem  TreatAsAtomicUnit=on
  Sport_Lv3_TqMap : Subsystem  TreatAsAtomicUnit=on
  Sport_Lv4_TqMap : Subsystem  TreatAsAtomicUnit=on
  Sport_Lv5_TqMap : Subsystem  TreatAsAtomicUnit=on
  Sport_OnePedal_TqMap : Subsystem  TreatAsAtomicUnit=on
  VTQD_WhlTqSPORTD_Nm : Outport
  wires:
  Equal6/1 -> If/6
  [VTQD_RegenMode_enum] -> Equal6/1
  Constant5/1 -> Equal6/2
  Equal5/1 -> If/5
  [VTQD_RegenMode_enum] -> Equal5/1
  Constant4/1 -> Equal5/2
  Equal4/1 -> If/4
  [VTQD_RegenMode_enum] -> Equal4/1
  Constant3/1 -> Equal4/2
  [VTQD_RegenMode_enum] -> Equal3/1
  Constant2/1 -> Equal3/2
  [VTQD_RegenMode_enum] -> Equal2/1
  Constant1/1 -> Equal2/2
  Constant/1 -> Equal1/2
  [VTQD_RegenMode_enum] -> Equal1/1
  [VTQD_SOPDTqMapD_Nm] -> Sport_OnePedal_TqMap/1(VTQD_SOPDTqMapDIn_Nm)
  If/6 -> Sport_OnePedal_TqMap/Action
  Sport_OnePedal_TqMap/1(VTQD_SOPDTqMapDOut_Nm) -> Merge/6
  [VTQD_SL5TqMapD_Nm] -> Sport_Lv5_TqMap/1(VTQD_SL5TqMapDIn_Nm)
  If/5 -> Sport_Lv5_TqMap/Action
  Sport_Lv5_TqMap/1(VTQD_SL5TqMapDOut_Nm) -> Merge/5
  Sport_Lv4_TqMap/1(VTQD_SL4TqMapDOut_Nm) -> Merge/4
  If/4 -> Sport_Lv4_TqMap/Action
  [VTQD_SL4TqMapD_Nm] -> Sport_Lv4_TqMap/1(VTQD_SL4TqMapDIn_Nm)
  [VTQD_SL3TqMapD_Nm] -> Sport_Lv3_TqMap/1(VTQD_SL3TqMapDIn_Nm)
  If/3 -> Sport_Lv3_TqMap/Action
  Sport_Lv3_TqMap/1(VTQD_SL3TqMapDOut_Nm) -> Merge/3
  [VTQD_SL2TqMapD_Nm] -> Sport_Lv2_TqMap/1(VTQD_SL2TqMapDIn_Nm)
  Sport_Lv2_TqMap/1(VTQD_SL2TqMapDOut_Nm) -> Merge/2
  If/2 -> Sport_Lv2_TqMap/Action
  Sport_Lv1_TqMap/1(VTQD_SL1TqMapDOut_Nm) -> Merge/1
  [VTQD_SL1TqMapD_Nm] -> Sport_Lv1_TqMap/1(VTQD_SL1TqMapDIn_Nm)
  Equal1/1 -> If/1
  Equal2/1 -> If/2
  If/1 -> Sport_Lv1_TqMap/Action
  Merge/1 -> VTQD_WhlTqSPORTD_Nm/1
  Equal3/1 -> If/3
  [VTQD_TqTargetShaftSpd_rpm] -> MTQD_SOPDTqMapD_Z_Nm/2
  [VTQD_ActAPSPosn_pct] -> MTQD_SOPDTqMapD_Z_Nm/1
  [VTQD_TqTargetShaftSpd_rpm] -> MTQD_SL5TqMapD_Z_Nm/2
  [VTQD_ActAPSPosn_pct] -> MTQD_SL5TqMapD_Z_Nm/1
  [VTQD_TqTargetShaftSpd_rpm] -> MTQD_SL3TqMapD_Z_Nm/2
  [VTQD_ActAPSPosn_pct] -> MTQD_SL3TqMapD_Z_Nm/1
  [VTQD_TqTargetShaftSpd_rpm] -> MTQD_SL2TqMapD_Z_Nm/2
  [VTQD_ActAPSPosn_pct] -> MTQD_SL2TqMapD_Z_Nm/1
  MTQD_SL5TqMapD_Z_Nm/1 -> [VTQD_SL5TqMapD_Nm]
  MTQD_SL4TqMapD_Z_Nm/1 -> [VTQD_SL4TqMapD_Nm]
  [VTQD_TqTargetShaftSpd_rpm] -> MTQD_SL4TqMapD_Z_Nm/2
  [VTQD_ActAPSPosn_pct] -> MTQD_SL4TqMapD_Z_Nm/1
  MTQD_SOPDTqMapD_Z_Nm/1 -> [VTQD_SOPDTqMapD_Nm]
  MTQD_SL3TqMapD_Z_Nm/1 -> [VTQD_SL3TqMapD_Nm]
  MTQD_SL2TqMapD_Z_Nm/1 -> [VTQD_SL2TqMapD_Nm]
  [VTQD_ActAPSPosn_pct] -> MTQD_SL1TqMapD_Z_Nm/1
  [VTQD_TqTargetShaftSpd_rpm] -> MTQD_SL1TqMapD_Z_Nm/2
  VTQD_RegenMode_enum/1 -> [VTQD_RegenMode_enum]
  VTQD_ActAPSPosn_pct/1 -> [VTQD_ActAPSPosn_pct]
  VTQD_TqTargetShaftSpd_rpm/1 -> [VTQD_TqTargetShaftSpd_rpm]
  MTQD_SL1TqMapD_Z_Nm/1 -> [VTQD_SL1TqMapD_Nm]
  [VTQD_SL1TqMapD_Nm] -> Sport_Invalid_TqMap1/1(VTQD_SL1TqMapDIn_Nm)
  If/7 -> Sport_Invalid_TqMap1/Action
  Sport_Invalid_TqMap1/1(VTQD_SL1TqMapDOut_Nm) -> Merge/7
  [VTQD_TqTargetShaftSpd_rpm] -> MTQD_SOPDTqMapDCon_Z_Nm/2
  [VVMC_EstSlope_Deg] -> MTQD_SOPDTqMapDCon_Z_Nm/1
  MTQD_SOPDTqMapDCon_Z_Nm/1 -> [VTQD_SOPDTqMapDCon_Nm]
  VVMC_EstSlope_Deg/1 -> [VVMC_EstSlope_Deg]
  VTQD_APSReqTimer_s/1 -> [VTQD_APSReqTimer_s]
  [VTQD_APSReqTimer_s] -> Sport_OnePedal_TqMap/3(VTQD_APSReqTimer_s)
  [VTQD_SOPDTqMapDCon_Nm] -> Sport_OnePedal_TqMap/2(VTQD_SOPDTqMapDCon_Nm)
  [VTQD_LowIdleAccPedal_flg] -> Sport_OnePedal_TqMap/4(VTQD_LowIdleAccPedal_flg)
  VTQD_LowIdleAccPedal_flg/1 -> [VTQD_LowIdleAccPedal_flg]
  VTQD_OPDHoldEnRel_flg/1 -> [VTQD_OPDHoldEnRel_flg]
  VTQD_VehActSpd_kph/1 -> [VTQD_VehActSpd_kph]
  VTQD_OPDHoldActRelTq_Nm/1 -> [VTQD_OPDHoldActRelTq_Nm]
  [VTQD_OPDHoldEnRel_flg] -> Sport_OnePedal_TqMap/5(VTQD_OPDHoldEnRel_flg)
  [VTQD_OPDHoldActRelTq_Nm] -> Sport_OnePedal_TqMap/6(VTQD_OPDHoldActRelTq_Nm)
  [VTQD_VehActSpd_kph] -> Sport_OnePedal_TqMap/7(VTQD_VehActSpd_kph)
  VTQD_SlopeUp_flg/1 -> [VTQD_SlopeUp_flg]
  [VTQD_SlopeUp_flg] -> Sport_OnePedal_TqMap/8(VTQD_SlopeUp_flg)
  RegenTqMapDComp_bus/1 -> [RegenTqMapDComp_bus]
  [RegenTqMapDComp_bus] -> Bus Selector/1
  Bus Selector/4 -> [VTQD_RL4TqMapDComp_Nm]  "<VTQD_RL4TqMapDComp_Nm>"
  Bus Selector/1 -> [VTQD_RL1TqMapDComp_Nm]  "<VTQD_RL1TqMapDComp_Nm>"
  Bus Selector/2 -> [VTQD_RL2TqMapDComp_Nm]  "<VTQD_RL2TqMapDComp_Nm>"
  Bus Selector/3 -> [VTQD_RL3TqMapDComp_Nm]  "<VTQD_RL3TqMapDComp_Nm>"
  Bus Selector/5 -> [VTQD_RL5TqMapDComp_Nm]  "<VTQD_RL5TqMapDComp_Nm>"
  [VTQD_RL1TqMapDComp_Nm] -> Sport_Lv1_TqMap/2(VTQD_RL1TqMapDComp_Nm)
  [VTQD_RL2TqMapDComp_Nm] -> Sport_Lv2_TqMap/2(VTQD_RL2TqMapDComp_Nm)
  [VTQD_RL3TqMapDComp_Nm] -> Sport_Lv3_TqMap/2(VTQD_RL3TqMapDComp_Nm)
  [VTQD_RL4TqMapDComp_Nm] -> Sport_Lv4_TqMap/2(VTQD_RL4TqMapDComp_Nm)
  [VTQD_RL5TqMapDComp_Nm] -> Sport_Lv5_TqMap/2(VTQD_RL5TqMapDComp_Nm)
  [VTQD_ActAPSPosn_pct] -> Sport_OnePedal_TqMap/9(VTQD_ActAPSPosn_pct1)

== system tqd/TQD/TorqueDemand/Signal_convert/SWC2_Subsystem/Big Mike Combo/Combo Key Detection/DiagnosisOff Mode/Key1/Maintain ==
  Input : Inport
  Action Port : ActionPort
  KeepKey1 : Outport
  wires:
  Input/1 -> KeepKey1/1

== system tqd/TQD/TorqueDemand/Signal_convert/SWC2_Subsystem/Big Mike Combo/Combo Key Detection/DiagnosisOff Mode/Key1/Reset ==
  Action Port : ActionPort
  Constant : Constant  Value=ENUM_COMBOKEY_NONE
  ResetToZero : Outport
  wires:
  Constant/1 -> ResetToZero/1

== system tqd/TQD/TorqueDemand/Signal_convert/SWC2_Subsystem/Big Mike Combo/Combo Key Detection/DiagnosisOff Mode/Key1/Write ==
  Input : Inport
  Action Port : ActionPort
  WriteCMD : Outport
  wires:
  Input/1 -> WriteCMD/1

== system tqd/TQD/TorqueDemand/Signal_convert/SWC2_Subsystem/Big Mike Combo/Combo Key Detection/DiagnosisOff Mode/Key2/Maintain ==
  Input : Inport
  Action Port : ActionPort
  KeepKey2 : Outport
  wires:
  Input/1 -> KeepKey2/1

== system tqd/TQD/TorqueDemand/Signal_convert/SWC2_Subsystem/Big Mike Combo/Combo Key Detection/DiagnosisOff Mode/Key2/Reset ==
  Action Port : ActionPort
  Constant : Constant  Value=ENUM_COMBOKEY_NONE
  ResetToZero : Outport
  wires:
  Constant/1 -> ResetToZero/1

== system tqd/TQD/TorqueDemand/Signal_convert/SWC2_Subsystem/Big Mike Combo/Combo Key Detection/DiagnosisOff Mode/Key2/Write ==
  Input : Inport
  Action Port : ActionPort
  WriteCMD : Outport
  wires:
  Input/1 -> WriteCMD/1

== system tqd/TQD/TorqueDemand/Signal_convert/SWC2_Subsystem/Big Mike Combo/Combo Key Detection/DiagnosisOff Mode/Key3/Maintain ==
  Input : Inport
  Action Port : ActionPort
  KeepKey3 : Outport
  wires:
  Input/1 -> KeepKey3/1

== system tqd/TQD/TorqueDemand/Signal_convert/SWC2_Subsystem/Big Mike Combo/Combo Key Detection/DiagnosisOff Mode/Key3/Reset ==
  Action Port : ActionPort
  Constant : Constant  Value=ENUM_COMBOKEY_NONE
  ResetToZero : Outport
  wires:
  Constant/1 -> ResetToZero/1

== system tqd/TQD/TorqueDemand/Signal_convert/SWC2_Subsystem/Big Mike Combo/Combo Key Detection/DiagnosisOff Mode/Key3/Write ==
  Input : Inport
  Action Port : ActionPort
  WriteCMD : Outport
  wires:
  Input/1 -> WriteCMD/1

== system tqd/TQD/TorqueDemand/Signal_convert/SWC2_Subsystem/Big Mike Combo/Combo Key Detection/DiagnosisOff Mode/Key4/Maintain ==
  Input : Inport
  Action Port : ActionPort
  KeepKey4 : Outport
  wires:
  Input/1 -> KeepKey4/1

== system tqd/TQD/TorqueDemand/Signal_convert/SWC2_Subsystem/Big Mike Combo/Combo Key Detection/DiagnosisOff Mode/Key4/Reset ==
  Action Port : ActionPort
  Constant : Constant  Value=ENUM_COMBOKEY_NONE
  ResetToZero : Outport
  wires:
  Constant/1 -> ResetToZero/1

== system tqd/TQD/TorqueDemand/Signal_convert/SWC2_Subsystem/Big Mike Combo/Combo Key Detection/DiagnosisOff Mode/Key4/Write ==
  Input : Inport
  Action Port : ActionPort
  WriteCMD : Outport
  wires:
  Input/1 -> WriteCMD/1

== system tqd/TQD/TorqueDemand/Signal_convert/SWC2_Subsystem/Big Mike Combo/Combo Key Detection/DiagnosisOff Mode/Key5/Maintain ==
  Input : Inport
  Action Port : ActionPort
  KeepKey5 : Outport
  wires:
  Input/1 -> KeepKey5/1

== system tqd/TQD/TorqueDemand/Signal_convert/SWC2_Subsystem/Big Mike Combo/Combo Key Detection/DiagnosisOff Mode/Key5/Reset ==
  Action Port : ActionPort
  Constant : Constant  Value=ENUM_COMBOKEY_NONE
  ResetToZero : Outport
  wires:
  Constant/1 -> ResetToZero/1

== system tqd/TQD/TorqueDemand/Signal_convert/SWC2_Subsystem/Big Mike Combo/Combo Key Detection/DiagnosisOff Mode/Key5/Write ==
  Input : Inport
  Action Port : ActionPort
  WriteCMD : Outport
  wires:
  Input/1 -> WriteCMD/1

== system tqd/TQD/TorqueDemand/Signal_convert/SWC2_Subsystem/Big Mike Combo/Combo Key Detection/DiagnosisOff Mode/Key6/Maintain ==
  Input : Inport
  Action Port : ActionPort
  KeepKey6 : Outport
  wires:
  Input/1 -> KeepKey6/1

== system tqd/TQD/TorqueDemand/Signal_convert/SWC2_Subsystem/Big Mike Combo/Combo Key Detection/DiagnosisOff Mode/Key6/Reset ==
  Action Port : ActionPort
  Constant : Constant  Value=ENUM_COMBOKEY_NONE
  ResetToZero : Outport
  wires:
  Constant/1 -> ResetToZero/1

== system tqd/TQD/TorqueDemand/Signal_convert/SWC2_Subsystem/Big Mike Combo/Combo Key Detection/DiagnosisOff Mode/Key6/Write ==
  Input : Inport
  Action Port : ActionPort
  WriteCMD : Outport
  wires:
  Input/1 -> WriteCMD/1

== system tqd/TQD/TorqueDemand/Signal_convert/SWC2_Subsystem/Big Mike Combo/Combo Key Detection/DiagnosisOff Mode/Key7/Maintain ==
  Input : Inport
  Action Port : ActionPort
  KeepKey7 : Outport
  wires:
  Input/1 -> KeepKey7/1

== system tqd/TQD/TorqueDemand/Signal_convert/SWC2_Subsystem/Big Mike Combo/Combo Key Detection/DiagnosisOff Mode/Key7/Reset ==
  Action Port : ActionPort
  Constant : Constant  Value=ENUM_COMBOKEY_NONE
  ResetToZero : Outport
  wires:
  Constant/1 -> ResetToZero/1

== system tqd/TQD/TorqueDemand/Signal_convert/SWC2_Subsystem/Big Mike Combo/Combo Key Detection/DiagnosisOff Mode/Key7/Write ==
  Input : Inport
  Action Port : ActionPort
  WriteCMD : Outport
  wires:
  Input/1 -> WriteCMD/1

== system tqd/TQD/TorqueDemand/Signal_convert/SWC2_Subsystem/Big Mike Combo/Combo Key Detection/DiagnosisOff Mode/Key8/Maintain ==
  Input : Inport
  Action Port : ActionPort
  KeepKey8 : Outport
  wires:
  Input/1 -> KeepKey8/1

== system tqd/TQD/TorqueDemand/Signal_convert/SWC2_Subsystem/Big Mike Combo/Combo Key Detection/DiagnosisOff Mode/Key8/Reset ==
  Action Port : ActionPort
  Constant : Constant  Value=ENUM_COMBOKEY_NONE
  ResetToZero : Outport
  wires:
  Constant/1 -> ResetToZero/1

== system tqd/TQD/TorqueDemand/Signal_convert/SWC2_Subsystem/Big Mike Combo/Combo Key Detection/DiagnosisOff Mode/Key8/Write ==
  Input : Inport
  Action Port : ActionPort
  WriteCMD : Outport
  wires:
  Input/1 -> WriteCMD/1

== system tqd/TQD/TorqueDemand/Signal_convert/SWC2_Subsystem/Big Mike Combo/Combo Key Detection/Engineering Mode/Key1/Maintain ==
  Input : Inport
  Action Port : ActionPort
  KeepKey1 : Outport
  wires:
  Input/1 -> KeepKey1/1

== system tqd/TQD/TorqueDemand/Signal_convert/SWC2_Subsystem/Big Mike Combo/Combo Key Detection/Engineering Mode/Key1/Reset ==
  Action Port : ActionPort
  Constant : Constant  Value=ENUM_COMBOKEY_NONE
  ResetToZero : Outport
  wires:
  Constant/1 -> ResetToZero/1

== system tqd/TQD/TorqueDemand/Signal_convert/SWC2_Subsystem/Big Mike Combo/Combo Key Detection/Engineering Mode/Key1/Write ==
  Input : Inport
  Action Port : ActionPort
  WriteCMD : Outport
  wires:
  Input/1 -> WriteCMD/1

== system tqd/TQD/TorqueDemand/Signal_convert/SWC2_Subsystem/Big Mike Combo/Combo Key Detection/Engineering Mode/Key2/Maintain ==
  Input : Inport
  Action Port : ActionPort
  KeepKey2 : Outport
  wires:
  Input/1 -> KeepKey2/1

== system tqd/TQD/TorqueDemand/Signal_convert/SWC2_Subsystem/Big Mike Combo/Combo Key Detection/Engineering Mode/Key2/Reset ==
  Action Port : ActionPort
  Constant : Constant  Value=ENUM_COMBOKEY_NONE
  ResetToZero : Outport
  wires:
  Constant/1 -> ResetToZero/1

== system tqd/TQD/TorqueDemand/Signal_convert/SWC2_Subsystem/Big Mike Combo/Combo Key Detection/Engineering Mode/Key2/Write ==
  Input : Inport
  Action Port : ActionPort
  WriteCMD : Outport
  wires:
  Input/1 -> WriteCMD/1

== system tqd/TQD/TorqueDemand/Signal_convert/SWC2_Subsystem/Big Mike Combo/Combo Key Detection/Engineering Mode/Key3/Maintain ==
  Input : Inport
  Action Port : ActionPort
  KeepKey3 : Outport
  wires:
  Input/1 -> KeepKey3/1

== system tqd/TQD/TorqueDemand/Signal_convert/SWC2_Subsystem/Big Mike Combo/Combo Key Detection/Engineering Mode/Key3/Reset ==
  Action Port : ActionPort
  Constant : Constant  Value=ENUM_COMBOKEY_NONE
  ResetToZero : Outport
  wires:
  Constant/1 -> ResetToZero/1

== system tqd/TQD/TorqueDemand/Signal_convert/SWC2_Subsystem/Big Mike Combo/Combo Key Detection/Engineering Mode/Key3/Write ==
  Input : Inport
  Action Port : ActionPort
  WriteCMD : Outport
  wires:
  Input/1 -> WriteCMD/1

== system tqd/TQD/TorqueDemand/Signal_convert/SWC2_Subsystem/Big Mike Combo/Combo Key Detection/Engineering Mode/Key4/Maintain ==
  Input : Inport
  Action Port : ActionPort
  KeepKey4 : Outport
  wires:
  Input/1 -> KeepKey4/1

== system tqd/TQD/TorqueDemand/Signal_convert/SWC2_Subsystem/Big Mike Combo/Combo Key Detection/Engineering Mode/Key4/Reset ==
  Action Port : ActionPort
  Constant : Constant  Value=ENUM_COMBOKEY_NONE
  ResetToZero : Outport
  wires:
  Constant/1 -> ResetToZero/1

== system tqd/TQD/TorqueDemand/Signal_convert/SWC2_Subsystem/Big Mike Combo/Combo Key Detection/Engineering Mode/Key4/Write ==
  Input : Inport
  Action Port : ActionPort
  WriteCMD : Outport
  wires:
  Input/1 -> WriteCMD/1

== system tqd/TQD/TorqueDemand/Signal_convert/SWC2_Subsystem/Big Mike Combo/Combo Key Detection/Engineering Mode/Key5/Maintain ==
  Input : Inport
  Action Port : ActionPort
  KeepKey5 : Outport
  wires:
  Input/1 -> KeepKey5/1

== system tqd/TQD/TorqueDemand/Signal_convert/SWC2_Subsystem/Big Mike Combo/Combo Key Detection/Engineering Mode/Key5/Reset ==
  Action Port : ActionPort
  Constant : Constant  Value=ENUM_COMBOKEY_NONE
  ResetToZero : Outport
  wires:
  Constant/1 -> ResetToZero/1

== system tqd/TQD/TorqueDemand/Signal_convert/SWC2_Subsystem/Big Mike Combo/Combo Key Detection/Engineering Mode/Key5/Write ==
  Input : Inport
  Action Port : ActionPort
  WriteCMD : Outport
  wires:
  Input/1 -> WriteCMD/1

== system tqd/TQD/TorqueDemand/Signal_convert/SWC2_Subsystem/Big Mike Combo/Combo Key Detection/Engineering Mode/Key6/Maintain ==
  Input : Inport
  Action Port : ActionPort
  KeepKey6 : Outport
  wires:
  Input/1 -> KeepKey6/1

== system tqd/TQD/TorqueDemand/Signal_convert/SWC2_Subsystem/Big Mike Combo/Combo Key Detection/Engineering Mode/Key6/Reset ==
  Action Port : ActionPort
  Constant : Constant  Value=ENUM_COMBOKEY_NONE
  ResetToZero : Outport
  wires:
  Constant/1 -> ResetToZero/1

== system tqd/TQD/TorqueDemand/Signal_convert/SWC2_Subsystem/Big Mike Combo/Combo Key Detection/Engineering Mode/Key6/Write ==
  Input : Inport
  Action Port : ActionPort
  WriteCMD : Outport
  wires:
  Input/1 -> WriteCMD/1

== system tqd/TQD/TorqueDemand/Signal_convert/SWC2_Subsystem/Big Mike Combo/Combo Key Detection/Engineering Mode/Key7/Maintain ==
  Input : Inport
  Action Port : ActionPort
  KeepKey7 : Outport
  wires:
  Input/1 -> KeepKey7/1

== system tqd/TQD/TorqueDemand/Signal_convert/SWC2_Subsystem/Big Mike Combo/Combo Key Detection/Engineering Mode/Key7/Reset ==
  Action Port : ActionPort
  Constant : Constant  Value=ENUM_COMBOKEY_NONE
  ResetToZero : Outport
  wires:
  Constant/1 -> ResetToZero/1

== system tqd/TQD/TorqueDemand/Signal_convert/SWC2_Subsystem/Big Mike Combo/Combo Key Detection/Engineering Mode/Key7/Write ==
  Input : Inport
  Action Port : ActionPort
  WriteCMD : Outport
  wires:
  Input/1 -> WriteCMD/1

== system tqd/TQD/TorqueDemand/Signal_convert/SWC2_Subsystem/Big Mike Combo/Combo Key Detection/Engineering Mode/Key8/Maintain ==
  Input : Inport
  Action Port : ActionPort
  KeepKey8 : Outport
  wires:
  Input/1 -> KeepKey8/1

== system tqd/TQD/TorqueDemand/Signal_convert/SWC2_Subsystem/Big Mike Combo/Combo Key Detection/Engineering Mode/Key8/Reset ==
  Action Port : ActionPort
  Constant : Constant  Value=ENUM_COMBOKEY_NONE
  ResetToZero : Outport
  wires:
  Constant/1 -> ResetToZero/1

== system tqd/TQD/TorqueDemand/Signal_convert/SWC2_Subsystem/Big Mike Combo/Combo Key Detection/Engineering Mode/Key8/Write ==
  Input : Inport
  Action Port : ActionPort
  WriteCMD : Outport
  wires:
  Input/1 -> WriteCMD/1

== system tqd/TQD/TorqueDemand/Signal_convert/SWC2_Subsystem/Big Mike Combo/Combo Key Detection/Exhibition Mode/Key1/Maintain ==
  Input : Inport
  Action Port : ActionPort
  KeepKey1 : Outport
  wires:
  Input/1 -> KeepKey1/1

== system tqd/TQD/TorqueDemand/Signal_convert/SWC2_Subsystem/Big Mike Combo/Combo Key Detection/Exhibition Mode/Key1/Reset ==
  Action Port : ActionPort
  Constant : Constant  Value=ENUM_COMBOKEY_NONE
  ResetToZero : Outport
  wires:
  Constant/1 -> ResetToZero/1

== system tqd/TQD/TorqueDemand/Signal_convert/SWC2_Subsystem/Big Mike Combo/Combo Key Detection/Exhibition Mode/Key1/Write ==
  Input : Inport
  Action Port : ActionPort
  WriteCMD : Outport
  wires:
  Input/1 -> WriteCMD/1

== system tqd/TQD/TorqueDemand/Signal_convert/SWC2_Subsystem/Big Mike Combo/Combo Key Detection/Exhibition Mode/Key2/Maintain ==
  Input : Inport
  Action Port : ActionPort
  KeepKey2 : Outport
  wires:
  Input/1 -> KeepKey2/1

== system tqd/TQD/TorqueDemand/Signal_convert/SWC2_Subsystem/Big Mike Combo/Combo Key Detection/Exhibition Mode/Key2/Reset ==
  Action Port : ActionPort
  Constant : Constant  Value=ENUM_COMBOKEY_NONE
  ResetToZero : Outport
  wires:
  Constant/1 -> ResetToZero/1

== system tqd/TQD/TorqueDemand/Signal_convert/SWC2_Subsystem/Big Mike Combo/Combo Key Detection/Exhibition Mode/Key2/Write ==
  Input : Inport
  Action Port : ActionPort
  WriteCMD : Outport
  wires:
  Input/1 -> WriteCMD/1

== system tqd/TQD/TorqueDemand/Signal_convert/SWC2_Subsystem/Big Mike Combo/Combo Key Detection/Exhibition Mode/Key3/Maintain ==
  Input : Inport
  Action Port : ActionPort
  KeepKey3 : Outport
  wires:
  Input/1 -> KeepKey3/1

== system tqd/TQD/TorqueDemand/Signal_convert/SWC2_Subsystem/Big Mike Combo/Combo Key Detection/Exhibition Mode/Key3/Reset ==
  Action Port : ActionPort
  Constant : Constant  Value=ENUM_COMBOKEY_NONE
  ResetToZero : Outport
  wires:
  Constant/1 -> ResetToZero/1

== system tqd/TQD/TorqueDemand/Signal_convert/SWC2_Subsystem/Big Mike Combo/Combo Key Detection/Exhibition Mode/Key3/Write ==
  Input : Inport
  Action Port : ActionPort
  WriteCMD : Outport
  wires:
  Input/1 -> WriteCMD/1

== system tqd/TQD/TorqueDemand/Signal_convert/SWC2_Subsystem/Big Mike Combo/Combo Key Detection/Exhibition Mode/Key4/Maintain ==
  Input : Inport
  Action Port : ActionPort
  KeepKey4 : Outport
  wires:
  Input/1 -> KeepKey4/1

== system tqd/TQD/TorqueDemand/Signal_convert/SWC2_Subsystem/Big Mike Combo/Combo Key Detection/Exhibition Mode/Key4/Reset ==
  Action Port : ActionPort
  Constant : Constant  Value=ENUM_COMBOKEY_NONE
  ResetToZero : Outport
  wires:
  Constant/1 -> ResetToZero/1

== system tqd/TQD/TorqueDemand/Signal_convert/SWC2_Subsystem/Big Mike Combo/Combo Key Detection/Exhibition Mode/Key4/Write ==
  Input : Inport
  Action Port : ActionPort
  WriteCMD : Outport
  wires:
  Input/1 -> WriteCMD/1

== system tqd/TQD/TorqueDemand/Signal_convert/SWC2_Subsystem/Big Mike Combo/Combo Key Detection/Exhibition Mode/Key5/Maintain ==
  Input : Inport
  Action Port : ActionPort
  KeepKey5 : Outport
  wires:
  Input/1 -> KeepKey5/1

== system tqd/TQD/TorqueDemand/Signal_convert/SWC2_Subsystem/Big Mike Combo/Combo Key Detection/Exhibition Mode/Key5/Reset ==
  Action Port : ActionPort
  Constant : Constant  Value=ENUM_COMBOKEY_NONE
  ResetToZero : Outport
  wires:
  Constant/1 -> ResetToZero/1

== system tqd/TQD/TorqueDemand/Signal_convert/SWC2_Subsystem/Big Mike Combo/Combo Key Detection/Exhibition Mode/Key5/Write ==
  Input : Inport
  Action Port : ActionPort
  WriteCMD : Outport
  wires:
  Input/1 -> WriteCMD/1

== system tqd/TQD/TorqueDemand/Signal_convert/SWC2_Subsystem/Big Mike Combo/Combo Key Detection/Exhibition Mode/Key6/Maintain ==
  Input : Inport
  Action Port : ActionPort
  KeepKey6 : Outport
  wires:
  Input/1 -> KeepKey6/1

== system tqd/TQD/TorqueDemand/Signal_convert/SWC2_Subsystem/Big Mike Combo/Combo Key Detection/Exhibition Mode/Key6/Reset ==
  Action Port : ActionPort
  Constant : Constant  Value=ENUM_COMBOKEY_NONE
  ResetToZero : Outport
  wires:
  Constant/1 -> ResetToZero/1

== system tqd/TQD/TorqueDemand/Signal_convert/SWC2_Subsystem/Big Mike Combo/Combo Key Detection/Exhibition Mode/Key6/Write ==
  Input : Inport
  Action Port : ActionPort
  WriteCMD : Outport
  wires:
  Input/1 -> WriteCMD/1

== system tqd/TQD/TorqueDemand/Signal_convert/SWC2_Subsystem/Big Mike Combo/Combo Key Detection/Exhibition Mode/Key7/Maintain ==
  Input : Inport
  Action Port : ActionPort
  KeepKey7 : Outport
  wires:
  Input/1 -> KeepKey7/1

== system tqd/TQD/TorqueDemand/Signal_convert/SWC2_Subsystem/Big Mike Combo/Combo Key Detection/Exhibition Mode/Key7/Reset ==
  Action Port : ActionPort
  Constant : Constant  Value=ENUM_COMBOKEY_NONE
  ResetToZero : Outport
  wires:
  Constant/1 -> ResetToZero/1

== system tqd/TQD/TorqueDemand/Signal_convert/SWC2_Subsystem/Big Mike Combo/Combo Key Detection/Exhibition Mode/Key7/Write ==
  Input : Inport
  Action Port : ActionPort
  WriteCMD : Outport
  wires:
  Input/1 -> WriteCMD/1

== system tqd/TQD/TorqueDemand/Signal_convert/SWC2_Subsystem/Big Mike Combo/Combo Key Detection/Exhibition Mode/Key8/Maintain ==
  Input : Inport
  Action Port : ActionPort
  KeepKey8 : Outport
  wires:
  Input/1 -> KeepKey8/1

== system tqd/TQD/TorqueDemand/Signal_convert/SWC2_Subsystem/Big Mike Combo/Combo Key Detection/Exhibition Mode/Key8/Reset ==
  Action Port : ActionPort
  Constant : Constant  Value=ENUM_COMBOKEY_NONE
  ResetToZero : Outport
  wires:
  Constant/1 -> ResetToZero/1

== system tqd/TQD/TorqueDemand/Signal_convert/SWC2_Subsystem/Big Mike Combo/Combo Key Detection/Exhibition Mode/Key8/Write ==
  Input : Inport
  Action Port : ActionPort
  WriteCMD : Outport
  wires:
  Input/1 -> WriteCMD/1

== system tqd/TQD/TorqueDemand/Signal_convert/SWC2_Subsystem/Big Mike Combo/Combo Key Detection/Manufacture Mode/Key1/Maintain ==
  Input : Inport
  Action Port : ActionPort
  KeepKey1 : Outport
  wires:
  Input/1 -> KeepKey1/1

== system tqd/TQD/TorqueDemand/Signal_convert/SWC2_Subsystem/Big Mike Combo/Combo Key Detection/Manufacture Mode/Key1/Reset ==
  Action Port : ActionPort
  Constant : Constant  Value=ENUM_COMBOKEY_NONE
  ResetToZero : Outport
  wires:
  Constant/1 -> ResetToZero/1

== system tqd/TQD/TorqueDemand/Signal_convert/SWC2_Subsystem/Big Mike Combo/Combo Key Detection/Manufacture Mode/Key1/Write ==
  Input : Inport
  Action Port : ActionPort
  WriteCMD : Outport
  wires:
  Input/1 -> WriteCMD/1

== system tqd/TQD/TorqueDemand/Signal_convert/SWC2_Subsystem/Big Mike Combo/Combo Key Detection/Manufacture Mode/Key2/Maintain ==
  Input : Inport
  Action Port : ActionPort
  KeepKey2 : Outport
  wires:
  Input/1 -> KeepKey2/1

== system tqd/TQD/TorqueDemand/Signal_convert/SWC2_Subsystem/Big Mike Combo/Combo Key Detection/Manufacture Mode/Key2/Reset ==
  Action Port : ActionPort
  Constant : Constant  Value=ENUM_COMBOKEY_NONE
  ResetToZero : Outport
  wires:
  Constant/1 -> ResetToZero/1

== system tqd/TQD/TorqueDemand/Signal_convert/SWC2_Subsystem/Big Mike Combo/Combo Key Detection/Manufacture Mode/Key2/Write ==
  Input : Inport
  Action Port : ActionPort
  WriteCMD : Outport
  wires:
  Input/1 -> WriteCMD/1

== system tqd/TQD/TorqueDemand/Signal_convert/SWC2_Subsystem/Big Mike Combo/Combo Key Detection/Manufacture Mode/Key3/Maintain ==
  Input : Inport
  Action Port : ActionPort
  KeepKey3 : Outport
  wires:
  Input/1 -> KeepKey3/1

== system tqd/TQD/TorqueDemand/Signal_convert/SWC2_Subsystem/Big Mike Combo/Combo Key Detection/Manufacture Mode/Key3/Reset ==
  Action Port : ActionPort
  Constant : Constant  Value=ENUM_COMBOKEY_NONE
  ResetToZero : Outport
  wires:
  Constant/1 -> ResetToZero/1

== system tqd/TQD/TorqueDemand/Signal_convert/SWC2_Subsystem/Big Mike Combo/Combo Key Detection/Manufacture Mode/Key3/Write ==
  Input : Inport
  Action Port : ActionPort
  WriteCMD : Outport
  wires:
  Input/1 -> WriteCMD/1

== system tqd/TQD/TorqueDemand/Signal_convert/SWC2_Subsystem/Big Mike Combo/Combo Key Detection/Manufacture Mode/Key4/Maintain ==
  Input : Inport
  Action Port : ActionPort
  KeepKey4 : Outport
  wires:
  Input/1 -> KeepKey4/1

== system tqd/TQD/TorqueDemand/Signal_convert/SWC2_Subsystem/Big Mike Combo/Combo Key Detection/Manufacture Mode/Key4/Reset ==
  Action Port : ActionPort
  Constant : Constant  Value=ENUM_COMBOKEY_NONE
  ResetToZero : Outport
  wires:
  Constant/1 -> ResetToZero/1

== system tqd/TQD/TorqueDemand/Signal_convert/SWC2_Subsystem/Big Mike Combo/Combo Key Detection/Manufacture Mode/Key4/Write ==
  Input : Inport
  Action Port : ActionPort
  WriteCMD : Outport
  wires:
  Input/1 -> WriteCMD/1
